simulink model "reference_model"  (R2019a)
settings: Solver=FixedStepAuto  StartTime=0.0  StopTime=10.0  FixedStep=0.1  RelTol=1e-3
InitFcn:
  | reference_model_init
values from neighbouring files (symbols this model uses):
  eta0 = [0,0,0,0,0,0]'    [init.m]
  nu0 = [0,0,0,0,0,0]'    [init.m]
  SimulationToRun = 5    [init.m]
undefined symbols (not defined in the file or in its folder): delta_refm, nu_dot_sat, nu_sat, omega_refm, useRefM
libraries: simulink x1
settings Model: Creator=Wai-Yen Chan  LastModifiedBy=den

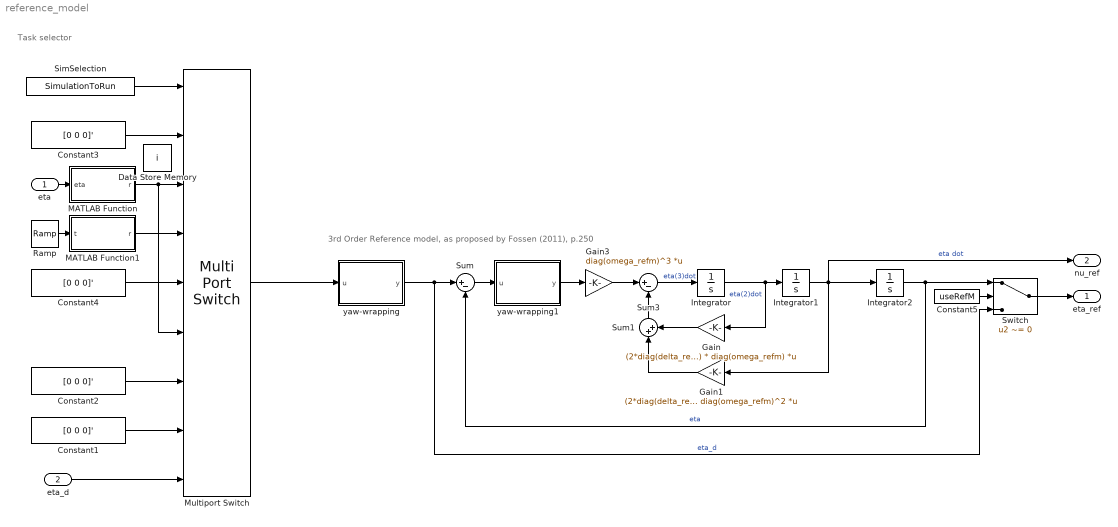
== system reference_model ==
  note: 3rd Order Reference model, as proposed by Fossen (2011), p.250
  note: Task selector
  eta : Inport  PortDimensions=3
  eta_d : Inport  Port=2  PortDimensions=3
  Constant{1..4} (4 alike) : Constant  Value=[0 0 0]'
  Constant5 : Constant  Value=useRefM
  Data Store Memory : DataStoreMemory  DataStoreName=i  InitialValue=1  ShowAdditionalParam=off  OutDataTypeStr=int8
  Gain : Gain  Gain=(2*diag(delta_refm)+eye(3)) * diag(omega_refm)  Multiplication=Matrix(K*u)
  Gain1 : Gain  Gain=(2*diag(delta_refm)+eye(3)) * diag(omega_refm)^2  Multiplication=Matrix(K*u)
  Gain3 : Gain  Gain=diag(omega_refm)^3  Multiplication=Matrix(K*u)
  Integrator : Integrator  LimitOutput=on  UpperSaturationLimit=nu_dot_sat  LowerSaturationLimit=-nu_dot_sat
  Integrator1 : Integrator  InitialCondition=[nu0(1:2)', nu0(6)]'  LimitOutput=on  UpperSaturationLimit=nu_sat  LowerSaturationLimit=-nu_sat
  Integrator2 : Integrator  InitialCondition=[eta0(1:2)', eta0(6)]'
  MATLAB Function : MATLAB Function  TreatAsAtomicUnit=on
  MATLAB Function1 : MATLAB Function  TreatAsAtomicUnit=on
  Multiport Switch : MultiPortSwitch  Inputs=8  DiagnosticForDefault=None
  Ramp : simulink/Sources/Ramp  slope=1  start=0  InitialOutput=0
  SimSelection : Constant  Value=SimulationToRun
  Sum : Sum  Inputs=|+-
  Sum1 : Sum  Inputs=|++
  Sum3 : Sum  Inputs=|+-
  Switch : Switch  Criteria=u2 ~= 0
  yaw-wrapping : MATLAB Function  TreatAsAtomicUnit=on
  yaw-wrapping1 : MATLAB Function  TreatAsAtomicUnit=on
  eta_ref : Outport  PortDimensions=3
  nu_ref : Outport  Port=2  PortDimensions=3
  wires:
  Multiport Switch/1 -> yaw-wrapping/1(u)
  Switch/1 -> eta_ref/1
  SimSelection/1 -> Multiport Switch/1
  Gain1/1 -> Sum1/1
  Integrator2/1 -> Sum/2, Switch/1  "eta"
  Constant3/1 -> Multiport Switch/2
  Sum3/1 -> Integrator/1  "eta(3)dot"
  Gain/1 -> Sum1/2
  Integrator/1 -> Gain/1, Integrator1/1  "eta(2)dot"
  Integrator1/1 -> Gain1/1, nu_ref/1, Integrator2/1  "eta dot"
  Constant5/1 -> Switch/2
  yaw-wrapping/1(y) -> Sum/1, Switch/3  "eta_d"
  eta/1 -> MATLAB Function/1(eta)
  MATLAB Function/1(r) -> Multiport Switch/6, Multiport Switch/3
  eta_d/1 -> Multiport Switch/9
  Constant1/1 -> Multiport Switch/8
  Constant2/1 -> Multiport Switch/7
  Constant4/1 -> Multiport Switch/5
  Sum1/1 -> Sum3/2
  Sum/1 -> yaw-wrapping1/1(u)
  Gain3/1 -> Sum3/1
  yaw-wrapping1/1(y) -> Gain3/1
  MATLAB Function1/1(r) -> Multiport Switch/4
  Ramp/1 -> MATLAB Function1/1(t)

== matlab function reference_model/yaw-wrapping ==
  data: u input; y output
function y = fcn(u)
    u(3) = mod(u(3)+pi, 2*pi) - pi; 
y = u;

== matlab function reference_model/yaw-wrapping1 ==
  data: u input; y output
function y = fcn(u)
    u(3) = mod(u(3)+pi, 2*pi) - pi; 
y = u;

== matlab function reference_model/MATLAB Function1 ==
  settings: updateMethod=DISCRETE
  data: r output; i data_store_memory; t input
function r = fcn(t)

ri = [ 0   0     0;
      50   0     0;
      50 -50     0;
      50 -50 -pi/4;
       0 -50 -pi/4;
       0   0     0 ]';

if t < 100
    r = ri(:,1);
elseif t < 400
    r = ri(:,2);
elseif t < 800
    r = ri(:,3);
elseif t < 1200
    r = ri(:,4);
elseif t < 1600
    r = ri(:,5);
else
    r = ri(:,6);
end

== matlab function reference_model/MATLAB Function ==
  settings: updateMethod=DISCRETE
  data: eta input; r output; i data_store_memory
function r = fcn(eta)

global i;
ri = [ 0   0     0;
      50   0     0;
      50 -50     0;
      50 -50 -pi/4;
       0 -50 -pi/4;
       0   0     0 ]';

if i ~= 6
    if (norm(eta(1:2)-ri(1:2,i)) < 0.2) && (abs(eta(3)-ri(3,i)) < 0.02)
        i = i + 1;
    end
end
   
r = ri(:,i);
